simulink model "FLIGHT_Hexacopter_fail"  (R2024a)
settings: Solver=FixedStepDiscrete  StartTime=0.0  StopTime=inf  FixedStep=SampleTime  RelTol=1e-3  EnableMultiTasking=on
InitFcn:
  | Init_FLIGHT_Hexacopter
values from neighbouring files (symbols this model uses):
  Kdpr = 0.004    [Init_FLIGHT_Hexacopter_fromNCMS.m]
  Kdrr = 0.004    [Init_FLIGHT_Hexacopter_fromNCMS.m]
  Kdvz = 0.0254    [Init_FLIGHT_Hexacopter_fromNCMS.m]
  Kdyr = 0.0298    [Init_FLIGHT_Hexacopter_fromNCMS.m]
  Kipr = 0.0    (= 0)    [Init_FLIGHT_Hexacopter_fromNCMS.m]
  Kirr = 0.0    (= 0)    [Init_FLIGHT_Hexacopter_fromNCMS.m]
  Kivz = 0.6304    [Init_FLIGHT_Hexacopter_fromNCMS.m]
  Kiyr = 0.0    (= 0)    [Init_FLIGHT_Hexacopter_fromNCMS.m]
  Kpp = 3.3894    [Init_FLIGHT_Hexacopter_fromNCMS.m]
  Kppr = 0.1    [Init_FLIGHT_Hexacopter_fromNCMS.m]
  Kpr = 3.3894    [Init_FLIGHT_Hexacopter_fromNCMS.m]
  Kprr = 0.1    [Init_FLIGHT_Hexacopter_fromNCMS.m]
  Kpvz = 0.3191    [Init_FLIGHT_Hexacopter_fromNCMS.m]
  Kpyr = 0.3744    [Init_FLIGHT_Hexacopter_fromNCMS.m]
  MAX_CONTROL_ANGLE_PITCH = 30*pi/180    (= 0.523598775598)    [Init_FLIGHT_Hexacopter.m]    (also in Init_FLIGHT_Hexacopter_fromNCMS.m = 0.349065850399)
  MAX_CONTROL_ANGLE_RATE_PITCH = 360*pi/180    (= 6.28318530718)    [Init_FLIGHT_Hexacopter.m]    (also in Init_FLIGHT_Hexacopter_fromNCMS.m)
  MAX_CONTROL_ANGLE_RATE_ROLL = 360*pi/180    (= 6.28318530718)    [Init_FLIGHT_Hexacopter.m]    (also in Init_FLIGHT_Hexacopter_fromNCMS.m)
  MAX_CONTROL_ANGLE_RATE_Y = 120*pi/180    (= 2.09439510239)    [Init_FLIGHT_Hexacopter.m]    (also in Init_FLIGHT_Hexacopter_fromNCMS.m)
  MAX_CONTROL_ANGLE_ROLL = 30*pi/180    (= 0.523598775598)    [Init_FLIGHT_Hexacopter.m]    (also in Init_FLIGHT_Hexacopter_fromNCMS.m = 0.349065850399)
  MAX_CONTROL_VELOCITY_Z = 1    [Init_FLIGHT_Hexacopter.m]    (also in Init_FLIGHT_Hexacopter_fromNCMS.m)
  Npr = 50    [Init_FLIGHT_Hexacopter_fromNCMS.m]
  Nrr = 50    [Init_FLIGHT_Hexacopter_fromNCMS.m]
  Nvz = Npr    (= 50)    [Init_FLIGHT_Hexacopter_fromNCMS.m]
  Nyr = 50    [Init_FLIGHT_Hexacopter_fromNCMS.m]
  SampleTime = 1/250    (= 0.004)    [Init_FLIGHT_Hexacopter.m]    (also in Init_FLIGHT_Hexacopter_fromNCMS.m = 0.01)
  THR_HOVER = 0.6085    [Init_FLIGHT_Hexacopter_fromNCMS.m]
libraries: px4lib x7, slpidlib x6, px4Sensorslib x3, simulink x2, px4uORBlib x1
(part 2 of 2)

== matlab function FLIGHT_Hexacopter_fail/Mixer/pwm_out2 ==
  data: Roll input; M1 output; Pitch input; Yaw input; Thrust input; M2 output; M3 output; M4 output; M5 output; M6 output
function [M1, M2, M3, M4, M5, M6] = motor_mixer(Roll, Pitch, Yaw, Thrust)
%Function description:
%  Control allocation. The quadrotor type is X-configuration,
%  and the airframe is as follows:
%3↓   1↑
 %  \ /
 %  / \
 %2↑   4↓
%Input：
%  Roll, Pitch, Yaw: attitude controller output.
%  Thrust

idle_PWM = 1000;
scale = 1000;
scale_att = scale*Thrust;

% M1 = uint16(Thrust*scale + (- Roll + Pitch + Yaw) * scale_att + idle_PWM);
% M2 = uint16(Thrust*scale + (Roll - Pitch + Yaw) * scale_att + idle_PWM);
% M3 = uint16(Thrust*scale + (Roll + Pitch - Yaw) * scale_att + idle_PWM);
% M4 = uint16(Thrust*scale + (- Roll - Pitch - Yaw) * scale_att + idle_PWM);

% Hex X (From Adam)
M1 = uint16(((-Roll - Yaw) * Thrust / 3 + Thrust) * 1000 + idle_PWM);
M2 = uint16(((Roll + Yaw) * Thrust / 3 + Thrust) * 1000 + idle_PWM);
M3 = uint16(((Pitch + (Roll / 2) - Yaw) * Thrust / 3 + Thrust) * 1000 + idle_PWM);
M4 = uint16(((-Pitch - (Roll / 2) + Yaw) * Thrust / 3 + Thrust) * 1000 + idle_PWM);
M5 = uint16(((Pitch - (Roll / 2) + Yaw) * Thrust / 3 + Thrust) * 1000 + idle_PWM);
M6 = uint16(((-Pitch + (Roll / 2) - Yaw) * Thrust / 3 + Thrust) * 1000 + idle_PWM);
